simulink model "AC_Overall"  (R2021b)
settings: Solver=VariableStepAuto  StartTime=0.0  StopTime=0.5  RelTol=1e-3
undefined symbols (not defined in the file): ac
libraries: acoustical_lib x129, nesl_utility x4
(part 2 of 3)

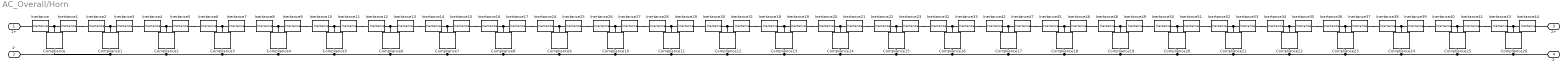
== system AC_Overall/Horn ==
  Compliance : acoustical_lib/Acoustical Elements/Compliance  c=ac.ho.C(1) m^3/Pa  r_c=1e-12 Pa/(m^3/s)  g_c=0 m^3/(Pa*s)  u_specify=off  u_priority=None  u=0 m^3/s  u_nominal_specify=off  u_nominal_unit=m^3/s  u_nominal_value=1  p_specify=off  p_priority=None  p=0 Pa  p_nominal_specify=off  p_nominal_unit=Pa  p_nominal_value=1  Pc_specify=off  Pc_priority=High  Pc=0 Pa  Pc_nominal_specify=off  Pc_nominal_unit=Pa  Pc_nominal_value=1
      settings: SourceProductName=Acoustical  InternalSimscapePortConfiguration="{\"Bottom\":[],\"Left\":[{\"id\":\"pp\",\"label\":\"+\",\"type\":\"acoustical.acoustical\"}],\"Right\":[{\"id\":\"nn\",\"label\":\"-\",\"type\":\"acoustical.acoustical\"}],\"Top\":[]}"
  Compliance1 : acoustical_lib/Acoustical Elements/Compliance  c=ac.ho.C(2) m^3/Pa  r_c=1e-12 Pa/(m^3/s)  g_c=0 m^3/(Pa*s)  u_specify=off  u_priority=None  u=0 m^3/s  u_nominal_specify=off  u_nominal_unit=m^3/s  u_nominal_value=1  p_specify=off  p_priority=None  p=0 Pa  p_nominal_specify=off  p_nominal_unit=Pa  p_nominal_value=1  Pc_specify=off  Pc_priority=High  Pc=0 Pa  Pc_nominal_specify=off  Pc_nominal_unit=Pa  Pc_nominal_value=1
      settings: SourceProductName=Acoustical  InternalSimscapePortConfiguration="{\"Bottom\":[],\"Left\":[{\"id\":\"pp\",\"label\":\"+\",\"type\":\"acoustical.acoustical\"}],\"Right\":[{\"id\":\"nn\",\"label\":\"-\",\"type\":\"acoustical.acoustical\"}],\"Top\":[]}"
  Compliance10 : acoustical_lib/Acoustical Elements/Compliance  c=ac.ho.C(11) m^3/Pa  r_c=1e-12 Pa/(m^3/s)  g_c=0 m^3/(Pa*s)  u_specify=off  u_priority=None  u=0 m^3/s  u_nominal_specify=off  u_nominal_unit=m^3/s  u_nominal_value=1  p_specify=off  p_priority=None  p=0 Pa  p_nominal_specify=off  p_nominal_unit=Pa  p_nominal_value=1  Pc_specify=off  Pc_priority=High  Pc=0 Pa  Pc_nominal_specify=off  Pc_nominal_unit=Pa  Pc_nominal_value=1
      settings: SourceProductName=Acoustical  InternalSimscapePortConfiguration="{\"Bottom\":[],\"Left\":[{\"id\":\"pp\",\"label\":\"+\",\"type\":\"acoustical.acoustical\"}],\"Right\":[{\"id\":\"nn\",\"label\":\"-\",\"type\":\"acoustical.acoustical\"}],\"Top\":[]}"
  Compliance11 : acoustical_lib/Acoustical Elements/Compliance  c=ac.ho.C(12) m^3/Pa  r_c=1e-12 Pa/(m^3/s)  g_c=0 m^3/(Pa*s)  u_specify=off  u_priority=None  u=0 m^3/s  u_nominal_specify=off  u_nominal_unit=m^3/s  u_nominal_value=1  p_specify=off  p_priority=None  p=0 Pa  p_nominal_specify=off  p_nominal_unit=Pa  p_nominal_value=1  Pc_specify=off  Pc_priority=High  Pc=0 Pa  Pc_nominal_specify=off  Pc_nominal_unit=Pa  Pc_nominal_value=1
      settings: SourceProductName=Acoustical  InternalSimscapePortConfiguration="{\"Bottom\":[],\"Left\":[{\"id\":\"pp\",\"label\":\"+\",\"type\":\"acoustical.acoustical\"}],\"Right\":[{\"id\":\"nn\",\"label\":\"-\",\"type\":\"acoustical.acoustical\"}],\"Top\":[]}"
  Compliance12 : acoustical_lib/Acoustical Elements/Compliance  c=ac.ho.C(13) m^3/Pa  r_c=1e-12 Pa/(m^3/s)  g_c=0 m^3/(Pa*s)  u_specify=off  u_priority=None  u=0 m^3/s  u_nominal_specify=off  u_nominal_unit=m^3/s  u_nominal_value=1  p_specify=off  p_priority=None  p=0 Pa  p_nominal_specify=off  p_nominal_unit=Pa  p_nominal_value=1  Pc_specify=off  Pc_priority=High  Pc=0 Pa  Pc_nominal_specify=off  Pc_nominal_unit=Pa  Pc_nominal_value=1
      settings: SourceProductName=Acoustical  InternalSimscapePortConfiguration="{\"Bottom\":[],\"Left\":[{\"id\":\"pp\",\"label\":\"+\",\"type\":\"acoustical.acoustical\"}],\"Right\":[{\"id\":\"nn\",\"label\":\"-\",\"type\":\"acoustical.acoustical\"}],\"Top\":[]}"
  Compliance13 : acoustical_lib/Acoustical Elements/Compliance  c=ac.ho.C(14) m^3/Pa  r_c=1e-12 Pa/(m^3/s)  g_c=0 m^3/(Pa*s)  u_specify=off  u_priority=None  u=0 m^3/s  u_nominal_specify=off  u_nominal_unit=m^3/s  u_nominal_value=1  p_specify=off  p_priority=None  p=0 Pa  p_nominal_specify=off  p_nominal_unit=Pa  p_nominal_value=1  Pc_specify=off  Pc_priority=High  Pc=0 Pa  Pc_nominal_specify=off  Pc_nominal_unit=Pa  Pc_nominal_value=1
      settings: SourceProductName=Acoustical  InternalSimscapePortConfiguration="{\"Bottom\":[],\"Left\":[{\"id\":\"pp\",\"label\":\"+\",\"type\":\"acoustical.acoustical\"}],\"Right\":[{\"id\":\"nn\",\"label\":\"-\",\"type\":\"acoustical.acoustical\"}],\"Top\":[]}"
  Compliance14 : acoustical_lib/Acoustical Elements/Compliance  c=ac.ho.C(15) m^3/Pa  r_c=1e-12 Pa/(m^3/s)  g_c=0 m^3/(Pa*s)  u_specify=off  u_priority=None  u=0 m^3/s  u_nominal_specify=off  u_nominal_unit=m^3/s  u_nominal_value=1  p_specify=off  p_priority=None  p=0 Pa  p_nominal_specify=off  p_nominal_unit=Pa  p_nominal_value=1  Pc_specify=off  Pc_priority=High  Pc=0 Pa  Pc_nominal_specify=off  Pc_nominal_unit=Pa  Pc_nominal_value=1
      settings: SourceProductName=Acoustical  InternalSimscapePortConfiguration="{\"Bottom\":[],\"Left\":[{\"id\":\"pp\",\"label\":\"+\",\"type\":\"acoustical.acoustical\"}],\"Right\":[{\"id\":\"nn\",\"label\":\"-\",\"type\":\"acoustical.acoustical\"}],\"Top\":[]}"
  Compliance15 : acoustical_lib/Acoustical Elements/Compliance  c=ac.ho.C(16) m^3/Pa  r_c=1e-12 Pa/(m^3/s)  g_c=0 m^3/(Pa*s)  u_specify=off  u_priority=None  u=0 m^3/s  u_nominal_specify=off  u_nominal_unit=m^3/s  u_nominal_value=1  p_specify=off  p_priority=None  p=0 Pa  p_nominal_specify=off  p_nominal_unit=Pa  p_nominal_value=1  Pc_specify=off  Pc_priority=High  Pc=0 Pa  Pc_nominal_specify=off  Pc_nominal_unit=Pa  Pc_nominal_value=1
      settings: SourceProductName=Acoustical  InternalSimscapePortConfiguration="{\"Bottom\":[],\"Left\":[{\"id\":\"pp\",\"label\":\"+\",\"type\":\"acoustical.acoustical\"}],\"Right\":[{\"id\":\"nn\",\"label\":\"-\",\"type\":\"acoustical.acoustical\"}],\"Top\":[]}"
  Compliance16 : acoustical_lib/Acoustical Elements/Compliance  c=ac.ho.C(17) m^3/Pa  r_c=1e-12 Pa/(m^3/s)  g_c=0 m^3/(Pa*s)  u_specify=off  u_priority=None  u=0 m^3/s  u_nominal_specify=off  u_nominal_unit=m^3/s  u_nominal_value=1  p_specify=off  p_priority=None  p=0 Pa  p_nominal_specify=off  p_nominal_unit=Pa  p_nominal_value=1  Pc_specify=off  Pc_priority=High  Pc=0 Pa  Pc_nominal_specify=off  Pc_nominal_unit=Pa  Pc_nominal_value=1
      settings: SourceProductName=Acoustical  InternalSimscapePortConfiguration="{\"Bottom\":[],\"Left\":[{\"id\":\"pp\",\"label\":\"+\",\"type\":\"acoustical.acoustical\"}],\"Right\":[{\"id\":\"nn\",\"label\":\"-\",\"type\":\"acoustical.acoustical\"}],\"Top\":[]}"
  Compliance17 : acoustical_lib/Acoustical Elements/Compliance  c=ac.ho.C(18) m^3/Pa  r_c=1e-12 Pa/(m^3/s)  g_c=0 m^3/(Pa*s)  u_specify=off  u_priority=None  u=0 m^3/s  u_nominal_specify=off  u_nominal_unit=m^3/s  u_nominal_value=1  p_specify=off  p_priority=None  p=0 Pa  p_nominal_specify=off  p_nominal_unit=Pa  p_nominal_value=1  Pc_specify=off  Pc_priority=High  Pc=0 Pa  Pc_nominal_specify=off  Pc_nominal_unit=Pa  Pc_nominal_value=1
      settings: SourceProductName=Acoustical  InternalSimscapePortConfiguration="{\"Bottom\":[],\"Left\":[{\"id\":\"pp\",\"label\":\"+\",\"type\":\"acoustical.acoustical\"}],\"Right\":[{\"id\":\"nn\",\"label\":\"-\",\"type\":\"acoustical.acoustical\"}],\"Top\":[]}"
  Compliance18 : acoustical_lib/Acoustical Elements/Compliance  c=ac.ho.C(19) m^3/Pa  r_c=1e-12 Pa/(m^3/s)  g_c=0 m^3/(Pa*s)  u_specify=off  u_priority=None  u=0 m^3/s  u_nominal_specify=off  u_nominal_unit=m^3/s  u_nominal_value=1  p_specify=off  p_priority=None  p=0 Pa  p_nominal_specify=off  p_nominal_unit=Pa  p_nominal_value=1  Pc_specify=off  Pc_priority=High  Pc=0 Pa  Pc_nominal_specify=off  Pc_nominal_unit=Pa  Pc_nominal_value=1
      settings: SourceProductName=Acoustical  InternalSimscapePortConfiguration="{\"Bottom\":[],\"Left\":[{\"id\":\"pp\",\"label\":\"+\",\"type\":\"acoustical.acoustical\"}],\"Right\":[{\"id\":\"nn\",\"label\":\"-\",\"type\":\"acoustical.acoustical\"}],\"Top\":[]}"
  Compliance19 : acoustical_lib/Acoustical Elements/Compliance  c=ac.ho.C(20) m^3/Pa  r_c=1e-12 Pa/(m^3/s)  g_c=0 m^3/(Pa*s)  u_specify=off  u_priority=None  u=0 m^3/s  u_nominal_specify=off  u_nominal_unit=m^3/s  u_nominal_value=1  p_specify=off  p_priority=None  p=0 Pa  p_nominal_specify=off  p_nominal_unit=Pa  p_nominal_value=1  Pc_specify=off  Pc_priority=High  Pc=0 Pa  Pc_nominal_specify=off  Pc_nominal_unit=Pa  Pc_nominal_value=1
      settings: SourceProductName=Acoustical  InternalSimscapePortConfiguration="{\"Bottom\":[],\"Left\":[{\"id\":\"pp\",\"label\":\"+\",\"type\":\"acoustical.acoustical\"}],\"Right\":[{\"id\":\"nn\",\"label\":\"-\",\"type\":\"acoustical.acoustical\"}],\"Top\":[]}"
  Compliance2 : acoustical_lib/Acoustical Elements/Compliance  c=ac.ho.C(3) m^3/Pa  r_c=1e-12 Pa/(m^3/s)  g_c=0 m^3/(Pa*s)  u_specify=off  u_priority=None  u=0 m^3/s  u_nominal_specify=off  u_nominal_unit=m^3/s  u_nominal_value=1  p_specify=off  p_priority=None  p=0 Pa  p_nominal_specify=off  p_nominal_unit=Pa  p_nominal_value=1  Pc_specify=off  Pc_priority=High  Pc=0 Pa  Pc_nominal_specify=off  Pc_nominal_unit=Pa  Pc_nominal_value=1
      settings: SourceProductName=Acoustical  InternalSimscapePortConfiguration="{\"Bottom\":[],\"Left\":[{\"id\":\"pp\",\"label\":\"+\",\"type\":\"acoustical.acoustical\"}],\"Right\":[{\"id\":\"nn\",\"label\":\"-\",\"type\":\"acoustical.acoustical\"}],\"Top\":[]}"
  Compliance20 : acoustical_lib/Acoustical Elements/Compliance  c=ac.ho.C(21) m^3/Pa  r_c=1e-12 Pa/(m^3/s)  g_c=0 m^3/(Pa*s)  u_specify=off  u_priority=None  u=0 m^3/s  u_nominal_specify=off  u_nominal_unit=m^3/s  u_nominal_value=1  p_specify=off  p_priority=None  p=0 Pa  p_nominal_specify=off  p_nominal_unit=Pa  p_nominal_value=1  Pc_specify=off  Pc_priority=High  Pc=0 Pa  Pc_nominal_specify=off  Pc_nominal_unit=Pa  Pc_nominal_value=1
      settings: SourceProductName=Acoustical  InternalSimscapePortConfiguration="{\"Bottom\":[],\"Left\":[{\"id\":\"pp\",\"label\":\"+\",\"type\":\"acoustical.acoustical\"}],\"Right\":[{\"id\":\"nn\",\"label\":\"-\",\"type\":\"acoustical.acoustical\"}],\"Top\":[]}"
  Compliance21 : acoustical_lib/Acoustical Elements/Compliance  c=ac.ho.C(22) m^3/Pa  r_c=1e-12 Pa/(m^3/s)  g_c=0 m^3/(Pa*s)  u_specify=off  u_priority=None  u=0 m^3/s  u_nominal_specify=off  u_nominal_unit=m^3/s  u_nominal_value=1  p_specify=off  p_priority=None  p=0 Pa  p_nominal_specify=off  p_nominal_unit=Pa  p_nominal_value=1  Pc_specify=off  Pc_priority=High  Pc=0 Pa  Pc_nominal_specify=off  Pc_nominal_unit=Pa  Pc_nominal_value=1
      settings: SourceProductName=Acoustical  InternalSimscapePortConfiguration="{\"Bottom\":[],\"Left\":[{\"id\":\"pp\",\"label\":\"+\",\"type\":\"acoustical.acoustical\"}],\"Right\":[{\"id\":\"nn\",\"label\":\"-\",\"type\":\"acoustical.acoustical\"}],\"Top\":[]}"
  Compliance22 : acoustical_lib/Acoustical Elements/Compliance  c=ac.ho.C(23) m^3/Pa  r_c=1e-12 Pa/(m^3/s)  g_c=0 m^3/(Pa*s)  u_specify=off  u_priority=None  u=0 m^3/s  u_nominal_specify=off  u_nominal_unit=m^3/s  u_nominal_value=1  p_specify=off  p_priority=None  p=0 Pa  p_nominal_specify=off  p_nominal_unit=Pa  p_nominal_value=1  Pc_specify=off  Pc_priority=High  Pc=0 Pa  Pc_nominal_specify=off  Pc_nominal_unit=Pa  Pc_nominal_value=1
      settings: SourceProductName=Acoustical  InternalSimscapePortConfiguration="{\"Bottom\":[],\"Left\":[{\"id\":\"pp\",\"label\":\"+\",\"type\":\"acoustical.acoustical\"}],\"Right\":[{\"id\":\"nn\",\"label\":\"-\",\"type\":\"acoustical.acoustical\"}],\"Top\":[]}"
  Compliance23 : acoustical_lib/Acoustical Elements/Compliance  c=ac.ho.C(24) m^3/Pa  r_c=1e-12 Pa/(m^3/s)  g_c=0 m^3/(Pa*s)  u_specify=off  u_priority=None  u=0 m^3/s  u_nominal_specify=off  u_nominal_unit=m^3/s  u_nominal_value=1  p_specify=off  p_priority=None  p=0 Pa  p_nominal_specify=off  p_nominal_unit=Pa  p_nominal_value=1  Pc_specify=off  Pc_priority=High  Pc=0 Pa  Pc_nominal_specify=off  Pc_nominal_unit=Pa  Pc_nominal_value=1
      settings: SourceProductName=Acoustical  InternalSimscapePortConfiguration="{\"Bottom\":[],\"Left\":[{\"id\":\"pp\",\"label\":\"+\",\"type\":\"acoustical.acoustical\"}],\"Right\":[{\"id\":\"nn\",\"label\":\"-\",\"type\":\"acoustical.acoustical\"}],\"Top\":[]}"
  Compliance24 : acoustical_lib/Acoustical Elements/Compliance  c=ac.ho.C(25) m^3/Pa  r_c=1e-12 Pa/(m^3/s)  g_c=0 m^3/(Pa*s)  u_specify=off  u_priority=None  u=0 m^3/s  u_nominal_specify=off  u_nominal_unit=m^3/s  u_nominal_value=1  p_specify=off  p_priority=None  p=0 Pa  p_nominal_specify=off  p_nominal_unit=Pa  p_nominal_value=1  Pc_specify=off  Pc_priority=High  Pc=0 Pa  Pc_nominal_specify=off  Pc_nominal_unit=Pa  Pc_nominal_value=1
      settings: SourceProductName=Acoustical  InternalSimscapePortConfiguration="{\"Bottom\":[],\"Left\":[{\"id\":\"pp\",\"label\":\"+\",\"type\":\"acoustical.acoustical\"}],\"Right\":[{\"id\":\"nn\",\"label\":\"-\",\"type\":\"acoustical.acoustical\"}],\"Top\":[]}"
  Compliance25 : acoustical_lib/Acoustical Elements/Compliance  c=ac.ho.C(26) m^3/Pa  r_c=1e-12 Pa/(m^3/s)  g_c=0 m^3/(Pa*s)  u_specify=off  u_priority=None  u=0 m^3/s  u_nominal_specify=off  u_nominal_unit=m^3/s  u_nominal_value=1  p_specify=off  p_priority=None  p=0 Pa  p_nominal_specify=off  p_nominal_unit=Pa  p_nominal_value=1  Pc_specify=off  Pc_priority=High  Pc=0 Pa  Pc_nominal_specify=off  Pc_nominal_unit=Pa  Pc_nominal_value=1
      settings: SourceProductName=Acoustical  InternalSimscapePortConfiguration="{\"Bottom\":[],\"Left\":[{\"id\":\"pp\",\"label\":\"+\",\"type\":\"acoustical.acoustical\"}],\"Right\":[{\"id\":\"nn\",\"label\":\"-\",\"type\":\"acoustical.acoustical\"}],\"Top\":[]}"
  Compliance26 : acoustical_lib/Acoustical Elements/Compliance  c=ac.ho.C(27) m^3/Pa  r_c=1e-12 Pa/(m^3/s)  g_c=0 m^3/(Pa*s)  u_specify=off  u_priority=None  u=0 m^3/s  u_nominal_specify=off  u_nominal_unit=m^3/s  u_nominal_value=1  p_specify=off  p_priority=None  p=0 Pa  p_nominal_specify=off  p_nominal_unit=Pa  p_nominal_value=1  Pc_specify=off  Pc_priority=High  Pc=0 Pa  Pc_nominal_specify=off  Pc_nominal_unit=Pa  Pc_nominal_value=1
      settings: SourceProductName=Acoustical  InternalSimscapePortConfiguration="{\"Bottom\":[],\"Left\":[{\"id\":\"pp\",\"label\":\"+\",\"type\":\"acoustical.acoustical\"}],\"Right\":[{\"id\":\"nn\",\"label\":\"-\",\"type\":\"acoustical.acoustical\"}],\"Top\":[]}"
  Compliance3 : acoustical_lib/Acoustical Elements/Compliance  c=ac.ho.C(4) m^3/Pa  r_c=1e-12 Pa/(m^3/s)  g_c=0 m^3/(Pa*s)  u_specify=off  u_priority=None  u=0 m^3/s  u_nominal_specify=off  u_nominal_unit=m^3/s  u_nominal_value=1  p_specify=off  p_priority=None  p=0 Pa  p_nominal_specify=off  p_nominal_unit=Pa  p_nominal_value=1  Pc_specify=off  Pc_priority=High  Pc=0 Pa  Pc_nominal_specify=off  Pc_nominal_unit=Pa  Pc_nominal_value=1
      settings: SourceProductName=Acoustical  InternalSimscapePortConfiguration="{\"Bottom\":[],\"Left\":[{\"id\":\"pp\",\"label\":\"+\",\"type\":\"acoustical.acoustical\"}],\"Right\":[{\"id\":\"nn\",\"label\":\"-\",\"type\":\"acoustical.acoustical\"}],\"Top\":[]}"
  Compliance4 : acoustical_lib/Acoustical Elements/Compliance  c=ac.ho.C(5) m^3/Pa  r_c=1e-12 Pa/(m^3/s)  g_c=0 m^3/(Pa*s)  u_specify=off  u_priority=None  u=0 m^3/s  u_nominal_specify=off  u_nominal_unit=m^3/s  u_nominal_value=1  p_specify=off  p_priority=None  p=0 Pa  p_nominal_specify=off  p_nominal_unit=Pa  p_nominal_value=1  Pc_specify=off  Pc_priority=High  Pc=0 Pa  Pc_nominal_specify=off  Pc_nominal_unit=Pa  Pc_nominal_value=1
      settings: SourceProductName=Acoustical  InternalSimscapePortConfiguration="{\"Bottom\":[],\"Left\":[{\"id\":\"pp\",\"label\":\"+\",\"type\":\"acoustical.acoustical\"}],\"Right\":[{\"id\":\"nn\",\"label\":\"-\",\"type\":\"acoustical.acoustical\"}],\"Top\":[]}"
  Compliance5 : acoustical_lib/Acoustical Elements/Compliance  c=ac.ho.C(6) m^3/Pa  r_c=1e-12 Pa/(m^3/s)  g_c=0 m^3/(Pa*s)  u_specify=off  u_priority=None  u=0 m^3/s  u_nominal_specify=off  u_nominal_unit=m^3/s  u_nominal_value=1  p_specify=off  p_priority=None  p=0 Pa  p_nominal_specify=off  p_nominal_unit=Pa  p_nominal_value=1  Pc_specify=off  Pc_priority=High  Pc=0 Pa  Pc_nominal_specify=off  Pc_nominal_unit=Pa  Pc_nominal_value=1
      settings: SourceProductName=Acoustical  InternalSimscapePortConfiguration="{\"Bottom\":[],\"Left\":[{\"id\":\"pp\",\"label\":\"+\",\"type\":\"acoustical.acoustical\"}],\"Right\":[{\"id\":\"nn\",\"label\":\"-\",\"type\":\"acoustical.acoustical\"}],\"Top\":[]}"
  Compliance6 : acoustical_lib/Acoustical Elements/Compliance  c=ac.ho.C(7) m^3/Pa  r_c=1e-12 Pa/(m^3/s)  g_c=0 m^3/(Pa*s)  u_specify=off  u_priority=None  u=0 m^3/s  u_nominal_specify=off  u_nominal_unit=m^3/s  u_nominal_value=1  p_specify=off  p_priority=None  p=0 Pa  p_nominal_specify=off  p_nominal_unit=Pa  p_nominal_value=1  Pc_specify=off  Pc_priority=High  Pc=0 Pa  Pc_nominal_specify=off  Pc_nominal_unit=Pa  Pc_nominal_value=1
      settings: SourceProductName=Acoustical  InternalSimscapePortConfiguration="{\"Bottom\":[],\"Left\":[{\"id\":\"pp\",\"label\":\"+\",\"type\":\"acoustical.acoustical\"}],\"Right\":[{\"id\":\"nn\",\"label\":\"-\",\"type\":\"acoustical.acoustical\"}],\"Top\":[]}"
  Compliance7 : acoustical_lib/Acoustical Elements/Compliance  c=ac.ho.C(8) m^3/Pa  r_c=1e-12 Pa/(m^3/s)  g_c=0 m^3/(Pa*s)  u_specify=off  u_priority=None  u=0 m^3/s  u_nominal_specify=off  u_nominal_unit=m^3/s  u_nominal_value=1  p_specify=off  p_priority=None  p=0 Pa  p_nominal_specify=off  p_nominal_unit=Pa  p_nominal_value=1  Pc_specify=off  Pc_priority=High  Pc=0 Pa  Pc_nominal_specify=off  Pc_nominal_unit=Pa  Pc_nominal_value=1
      settings: SourceProductName=Acoustical  InternalSimscapePortConfiguration="{\"Bottom\":[],\"Left\":[{\"id\":\"pp\",\"label\":\"+\",\"type\":\"acoustical.acoustical\"}],\"Right\":[{\"id\":\"nn\",\"label\":\"-\",\"type\":\"acoustical.acoustical\"}],\"Top\":[]}"
  Compliance8 : acoustical_lib/Acoustical Elements/Compliance  c=ac.ho.C(9) m^3/Pa  r_c=1e-12 Pa/(m^3/s)  g_c=0 m^3/(Pa*s)  u_specify=off  u_priority=None  u=0 m^3/s  u_nominal_specify=off  u_nominal_unit=m^3/s  u_nominal_value=1  p_specify=off  p_priority=None  p=0 Pa  p_nominal_specify=off  p_nominal_unit=Pa  p_nominal_value=1  Pc_specify=off  Pc_priority=High  Pc=0 Pa  Pc_nominal_specify=off  Pc_nominal_unit=Pa  Pc_nominal_value=1
      settings: SourceProductName=Acoustical  InternalSimscapePortConfiguration="{\"Bottom\":[],\"Left\":[{\"id\":\"pp\",\"label\":\"+\",\"type\":\"acoustical.acoustical\"}],\"Right\":[{\"id\":\"nn\",\"label\":\"-\",\"type\":\"acoustical.acoustical\"}],\"Top\":[]}"
  Compliance9 : acoustical_lib/Acoustical Elements/Compliance  c=ac.ho.C(10) m^3/Pa  r_c=1e-12 Pa/(m^3/s)  g_c=0 m^3/(Pa*s)  u_specify=off  u_priority=None  u=0 m^3/s  u_nominal_specify=off  u_nominal_unit=m^3/s  u_nominal_value=1  p_specify=off  p_priority=None  p=0 Pa  p_nominal_specify=off  p_nominal_unit=Pa  p_nominal_value=1  Pc_specify=off  Pc_priority=High  Pc=0 Pa  Pc_nominal_specify=off  Pc_nominal_unit=Pa  Pc_nominal_value=1
      settings: SourceProductName=Acoustical  InternalSimscapePortConfiguration="{\"Bottom\":[],\"Left\":[{\"id\":\"pp\",\"label\":\"+\",\"type\":\"acoustical.acoustical\"}],\"Right\":[{\"id\":\"nn\",\"label\":\"-\",\"type\":\"acoustical.acoustical\"}],\"Top\":[]}"
  Inertance : acoustical_lib/Acoustical Elements/Inertance  m=ac.ho.L(1) Pa*s^2/m^3  r_m=0 Pa/(m^3/s)  g_m=1e-12 m^3/(Pa*s)  u_specify=off  u_priority=None  u=0 m^3/s  u_nominal_specify=off  u_nominal_unit=m^3/s  u_nominal_value=1  p_specify=off  p_priority=None  p=0 Pa  p_nominal_specify=off  p_nominal_unit=Pa  p_nominal_value=1  U_m_specify=off  U_m_priority=High  U_m=0 m^3/s  U_m_nominal_specify=off  U_m_nominal_unit=m^3/s  U_m_nominal_value=1
      settings: SourceProductName=Acoustical  InternalSimscapePortConfiguration="{\"Bottom\":[],\"Left\":[{\"id\":\"pp\",\"label\":\"+\",\"type\":\"acoustical.acoustical\"}],\"Right\":[{\"id\":\"nn\",\"label\":\"-\",\"type\":\"acoustical.acoustical\"}],\"Top\":[]}"
  Inertance1 : acoustical_lib/Acoustical Elements/Inertance  m=ac.ho.L(1) Pa*s^2/m^3  r_m=0 Pa/(m^3/s)  g_m=1e-12 m^3/(Pa*s)  u_specify=off  u_priority=None  u=0 m^3/s  u_nominal_specify=off  u_nominal_unit=m^3/s  u_nominal_value=1  p_specify=off  p_priority=None  p=0 Pa  p_nominal_specify=off  p_nominal_unit=Pa  p_nominal_value=1  U_m_specify=off  U_m_priority=High  U_m=0 m^3/s  U_m_nominal_specify=off  U_m_nominal_unit=m^3/s  U_m_nominal_value=1
      settings: SourceProductName=Acoustical  InternalSimscapePortConfiguration="{\"Bottom\":[],\"Left\":[{\"id\":\"pp\",\"label\":\"+\",\"type\":\"acoustical.acoustical\"}],\"Right\":[{\"id\":\"nn\",\"label\":\"-\",\"type\":\"acoustical.acoustical\"}],\"Top\":[]}"
  Inertance10 : acoustical_lib/Acoustical Elements/Inertance  m=ac.ho.L(6) Pa*s^2/m^3  r_m=0 Pa/(m^3/s)  g_m=1e-12 m^3/(Pa*s)  u_specify=off  u_priority=None  u=0 m^3/s  u_nominal_specify=off  u_nominal_unit=m^3/s  u_nominal_value=1  p_specify=off  p_priority=None  p=0 Pa  p_nominal_specify=off  p_nominal_unit=Pa  p_nominal_value=1  U_m_specify=off  U_m_priority=High  U_m=0 m^3/s  U_m_nominal_specify=off  U_m_nominal_unit=m^3/s  U_m_nominal_value=1
      settings: SourceProductName=Acoustical  InternalSimscapePortConfiguration="{\"Bottom\":[],\"Left\":[{\"id\":\"pp\",\"label\":\"+\",\"type\":\"acoustical.acoustical\"}],\"Right\":[{\"id\":\"nn\",\"label\":\"-\",\"type\":\"acoustical.acoustical\"}],\"Top\":[]}"
  Inertance11 : acoustical_lib/Acoustical Elements/Inertance  m=ac.ho.L(6) Pa*s^2/m^3  r_m=0 Pa/(m^3/s)  g_m=1e-12 m^3/(Pa*s)  u_specify=off  u_priority=None  u=0 m^3/s  u_nominal_specify=off  u_nominal_unit=m^3/s  u_nominal_value=1  p_specify=off  p_priority=None  p=0 Pa  p_nominal_specify=off  p_nominal_unit=Pa  p_nominal_value=1  U_m_specify=off  U_m_priority=High  U_m=0 m^3/s  U_m_nominal_specify=off  U_m_nominal_unit=m^3/s  U_m_nominal_value=1
      settings: SourceProductName=Acoustical  InternalSimscapePortConfiguration="{\"Bottom\":[],\"Left\":[{\"id\":\"pp\",\"label\":\"+\",\"type\":\"acoustical.acoustical\"}],\"Right\":[{\"id\":\"nn\",\"label\":\"-\",\"type\":\"acoustical.acoustical\"}],\"Top\":[]}"
  Inertance12 : acoustical_lib/Acoustical Elements/Inertance  m=ac.ho.L(7) Pa*s^2/m^3  r_m=0 Pa/(m^3/s)  g_m=1e-12 m^3/(Pa*s)  u_specify=off  u_priority=None  u=0 m^3/s  u_nominal_specify=off  u_nominal_unit=m^3/s  u_nominal_value=1  p_specify=off  p_priority=None  p=0 Pa  p_nominal_specify=off  p_nominal_unit=Pa  p_nominal_value=1  U_m_specify=off  U_m_priority=High  U_m=0 m^3/s  U_m_nominal_specify=off  U_m_nominal_unit=m^3/s  U_m_nominal_value=1
      settings: SourceProductName=Acoustical  InternalSimscapePortConfiguration="{\"Bottom\":[],\"Left\":[{\"id\":\"pp\",\"label\":\"+\",\"type\":\"acoustical.acoustical\"}],\"Right\":[{\"id\":\"nn\",\"label\":\"-\",\"type\":\"acoustical.acoustical\"}],\"Top\":[]}"
  Inertance13 : acoustical_lib/Acoustical Elements/Inertance  m=ac.ho.L(7) Pa*s^2/m^3  r_m=0 Pa/(m^3/s)  g_m=1e-12 m^3/(Pa*s)  u_specify=off  u_priority=None  u=0 m^3/s  u_nominal_specify=off  u_nominal_unit=m^3/s  u_nominal_value=1  p_specify=off  p_priority=None  p=0 Pa  p_nominal_specify=off  p_nominal_unit=Pa  p_nominal_value=1  U_m_specify=off  U_m_priority=High  U_m=0 m^3/s  U_m_nominal_specify=off  U_m_nominal_unit=m^3/s  U_m_nominal_value=1
      settings: SourceProductName=Acoustical  InternalSimscapePortConfiguration="{\"Bottom\":[],\"Left\":[{\"id\":\"pp\",\"label\":\"+\",\"type\":\"acoustical.acoustical\"}],\"Right\":[{\"id\":\"nn\",\"label\":\"-\",\"type\":\"acoustical.acoustical\"}],\"Top\":[]}"
  Inertance14 : acoustical_lib/Acoustical Elements/Inertance  m=ac.ho.L(8) Pa*s^2/m^3  r_m=0 Pa/(m^3/s)  g_m=1e-12 m^3/(Pa*s)  u_specify=off  u_priority=None  u=0 m^3/s  u_nominal_specify=off  u_nominal_unit=m^3/s  u_nominal_value=1  p_specify=off  p_priority=None  p=0 Pa  p_nominal_specify=off  p_nominal_unit=Pa  p_nominal_value=1  U_m_specify=off  U_m_priority=High  U_m=0 m^3/s  U_m_nominal_specify=off  U_m_nominal_unit=m^3/s  U_m_nominal_value=1
      settings: SourceProductName=Acoustical  InternalSimscapePortConfiguration="{\"Bottom\":[],\"Left\":[{\"id\":\"pp\",\"label\":\"+\",\"type\":\"acoustical.acoustical\"}],\"Right\":[{\"id\":\"nn\",\"label\":\"-\",\"type\":\"acoustical.acoustical\"}],\"Top\":[]}"
  Inertance15 : acoustical_lib/Acoustical Elements/Inertance  m=ac.ho.L(8) Pa*s^2/m^3  r_m=0 Pa/(m^3/s)  g_m=1e-12 m^3/(Pa*s)  u_specify=off  u_priority=None  u=0 m^3/s  u_nominal_specify=off  u_nominal_unit=m^3/s  u_nominal_value=1  p_specify=off  p_priority=None  p=0 Pa  p_nominal_specify=off  p_nominal_unit=Pa  p_nominal_value=1  U_m_specify=off  U_m_priority=High  U_m=0 m^3/s  U_m_nominal_specify=off  U_m_nominal_unit=m^3/s  U_m_nominal_value=1
      settings: SourceProductName=Acoustical  InternalSimscapePortConfiguration="{\"Bottom\":[],\"Left\":[{\"id\":\"pp\",\"label\":\"+\",\"type\":\"acoustical.acoustical\"}],\"Right\":[{\"id\":\"nn\",\"label\":\"-\",\"type\":\"acoustical.acoustical\"}],\"Top\":[]}"
  Inertance16 : acoustical_lib/Acoustical Elements/Inertance  m=ac.ho.L(9) Pa*s^2/m^3  r_m=0 Pa/(m^3/s)  g_m=1e-12 m^3/(Pa*s)  u_specify=off  u_priority=None  u=0 m^3/s  u_nominal_specify=off  u_nominal_unit=m^3/s  u_nominal_value=1  p_specify=off  p_priority=None  p=0 Pa  p_nominal_specify=off  p_nominal_unit=Pa  p_nominal_value=1  U_m_specify=off  U_m_priority=High  U_m=0 m^3/s  U_m_nominal_specify=off  U_m_nominal_unit=m^3/s  U_m_nominal_value=1
      settings: SourceProductName=Acoustical  InternalSimscapePortConfiguration="{\"Bottom\":[],\"Left\":[{\"id\":\"pp\",\"label\":\"+\",\"type\":\"acoustical.acoustical\"}],\"Right\":[{\"id\":\"nn\",\"label\":\"-\",\"type\":\"acoustical.acoustical\"}],\"Top\":[]}"
  Inertance17 : acoustical_lib/Acoustical Elements/Inertance  m=ac.ho.L(9) Pa*s^2/m^3  r_m=0 Pa/(m^3/s)  g_m=1e-12 m^3/(Pa*s)  u_specify=off  u_priority=None  u=0 m^3/s  u_nominal_specify=off  u_nominal_unit=m^3/s  u_nominal_value=1  p_specify=off  p_priority=None  p=0 Pa  p_nominal_specify=off  p_nominal_unit=Pa  p_nominal_value=1  U_m_specify=off  U_m_priority=High  U_m=0 m^3/s  U_m_nominal_specify=off  U_m_nominal_unit=m^3/s  U_m_nominal_value=1
      settings: SourceProductName=Acoustical  InternalSimscapePortConfiguration="{\"Bottom\":[],\"Left\":[{\"id\":\"pp\",\"label\":\"+\",\"type\":\"acoustical.acoustical\"}],\"Right\":[{\"id\":\"nn\",\"label\":\"-\",\"type\":\"acoustical.acoustical\"}],\"Top\":[]}"
  Inertance18 : acoustical_lib/Acoustical Elements/Inertance  m=ac.ho.L(14) Pa*s^2/m^3  r_m=0 Pa/(m^3/s)  g_m=1e-12 m^3/(Pa*s)  u_specify=off  u_priority=None  u=0 m^3/s  u_nominal_specify=off  u_nominal_unit=m^3/s  u_nominal_value=1  p_specify=off  p_priority=None  p=0 Pa  p_nominal_specify=off  p_nominal_unit=Pa  p_nominal_value=1  U_m_specify=off  U_m_priority=High  U_m=0 m^3/s  U_m_nominal_specify=off  U_m_nominal_unit=m^3/s  U_m_nominal_value=1
      settings: SourceProductName=Acoustical  InternalSimscapePortConfiguration="{\"Bottom\":[],\"Left\":[{\"id\":\"pp\",\"label\":\"+\",\"type\":\"acoustical.acoustical\"}],\"Right\":[{\"id\":\"nn\",\"label\":\"-\",\"type\":\"acoustical.acoustical\"}],\"Top\":[]}"
  Inertance19 : acoustical_lib/Acoustical Elements/Inertance  m=ac.ho.L(14) Pa*s^2/m^3  r_m=0 Pa/(m^3/s)  g_m=1e-12 m^3/(Pa*s)  u_specify=off  u_priority=None  u=0 m^3/s  u_nominal_specify=off  u_nominal_unit=m^3/s  u_nominal_value=1  p_specify=off  p_priority=None  p=0 Pa  p_nominal_specify=off  p_nominal_unit=Pa  p_nominal_value=1  U_m_specify=off  U_m_priority=High  U_m=0 m^3/s  U_m_nominal_specify=off  U_m_nominal_unit=m^3/s  U_m_nominal_value=1
      settings: SourceProductName=Acoustical  InternalSimscapePortConfiguration="{\"Bottom\":[],\"Left\":[{\"id\":\"pp\",\"label\":\"+\",\"type\":\"acoustical.acoustical\"}],\"Right\":[{\"id\":\"nn\",\"label\":\"-\",\"type\":\"acoustical.acoustical\"}],\"Top\":[]}"
  Inertance2 : acoustical_lib/Acoustical Elements/Inertance  m=ac.ho.L(2) Pa*s^2/m^3  r_m=0 Pa/(m^3/s)  g_m=1e-12 m^3/(Pa*s)  u_specify=off  u_priority=None  u=0 m^3/s  u_nominal_specify=off  u_nominal_unit=m^3/s  u_nominal_value=1  p_specify=off  p_priority=None  p=0 Pa  p_nominal_specify=off  p_nominal_unit=Pa  p_nominal_value=1  U_m_specify=off  U_m_priority=High  U_m=0 m^3/s  U_m_nominal_specify=off  U_m_nominal_unit=m^3/s  U_m_nominal_value=1
      settings: SourceProductName=Acoustical  InternalSimscapePortConfiguration="{\"Bottom\":[],\"Left\":[{\"id\":\"pp\",\"label\":\"+\",\"type\":\"acoustical.acoustical\"}],\"Right\":[{\"id\":\"nn\",\"label\":\"-\",\"type\":\"acoustical.acoustical\"}],\"Top\":[]}"
  Inertance20 : acoustical_lib/Acoustical Elements/Inertance  m=ac.ho.L(15) Pa*s^2/m^3  r_m=0 Pa/(m^3/s)  g_m=1e-12 m^3/(Pa*s)  u_specify=off  u_priority=None  u=0 m^3/s  u_nominal_specify=off  u_nominal_unit=m^3/s  u_nominal_value=1  p_specify=off  p_priority=None  p=0 Pa  p_nominal_specify=off  p_nominal_unit=Pa  p_nominal_value=1  U_m_specify=off  U_m_priority=High  U_m=0 m^3/s  U_m_nominal_specify=off  U_m_nominal_unit=m^3/s  U_m_nominal_value=1
      settings: SourceProductName=Acoustical  InternalSimscapePortConfiguration="{\"Bottom\":[],\"Left\":[{\"id\":\"pp\",\"label\":\"+\",\"type\":\"acoustical.acoustical\"}],\"Right\":[{\"id\":\"nn\",\"label\":\"-\",\"type\":\"acoustical.acoustical\"}],\"Top\":[]}"
  Inertance21 : acoustical_lib/Acoustical Elements/Inertance  m=ac.ho.L(15) Pa*s^2/m^3  r_m=0 Pa/(m^3/s)  g_m=1e-12 m^3/(Pa*s)  u_specify=off  u_priority=None  u=0 m^3/s  u_nominal_specify=off  u_nominal_unit=m^3/s  u_nominal_value=1  p_specify=off  p_priority=None  p=0 Pa  p_nominal_specify=off  p_nominal_unit=Pa  p_nominal_value=1  U_m_specify=off  U_m_priority=High  U_m=0 m^3/s  U_m_nominal_specify=off  U_m_nominal_unit=m^3/s  U_m_nominal_value=1
      settings: SourceProductName=Acoustical  InternalSimscapePortConfiguration="{\"Bottom\":[],\"Left\":[{\"id\":\"pp\",\"label\":\"+\",\"type\":\"acoustical.acoustical\"}],\"Right\":[{\"id\":\"nn\",\"label\":\"-\",\"type\":\"acoustical.acoustical\"}],\"Top\":[]}"
  Inertance22 : acoustical_lib/Acoustical Elements/Inertance  m=ac.ho.L(16) Pa*s^2/m^3  r_m=0 Pa/(m^3/s)  g_m=1e-12 m^3/(Pa*s)  u_specify=off  u_priority=None  u=0 m^3/s  u_nominal_specify=off  u_nominal_unit=m^3/s  u_nominal_value=1  p_specify=off  p_priority=None  p=0 Pa  p_nominal_specify=off  p_nominal_unit=Pa  p_nominal_value=1  U_m_specify=off  U_m_priority=High  U_m=0 m^3/s  U_m_nominal_specify=off  U_m_nominal_unit=m^3/s  U_m_nominal_value=1
      settings: SourceProductName=Acoustical  InternalSimscapePortConfiguration="{\"Bottom\":[],\"Left\":[{\"id\":\"pp\",\"label\":\"+\",\"type\":\"acoustical.acoustical\"}],\"Right\":[{\"id\":\"nn\",\"label\":\"-\",\"type\":\"acoustical.acoustical\"}],\"Top\":[]}"
  Inertance23 : acoustical_lib/Acoustical Elements/Inertance  m=ac.ho.L(16) Pa*s^2/m^3  r_m=0 Pa/(m^3/s)  g_m=1e-12 m^3/(Pa*s)  u_specify=off  u_priority=None  u=0 m^3/s  u_nominal_specify=off  u_nominal_unit=m^3/s  u_nominal_value=1  p_specify=off  p_priority=None  p=0 Pa  p_nominal_specify=off  p_nominal_unit=Pa  p_nominal_value=1  U_m_specify=off  U_m_priority=High  U_m=0 m^3/s  U_m_nominal_specify=off  U_m_nominal_unit=m^3/s  U_m_nominal_value=1
      settings: SourceProductName=Acoustical  InternalSimscapePortConfiguration="{\"Bottom\":[],\"Left\":[{\"id\":\"pp\",\"label\":\"+\",\"type\":\"acoustical.acoustical\"}],\"Right\":[{\"id\":\"nn\",\"label\":\"-\",\"type\":\"acoustical.acoustical\"}],\"Top\":[]}"
  Inertance24 : acoustical_lib/Acoustical Elements/Inertance  m=ac.ho.L(10) Pa*s^2/m^3  r_m=0 Pa/(m^3/s)  g_m=1e-12 m^3/(Pa*s)  u_specify=off  u_priority=None  u=0 m^3/s  u_nominal_specify=off  u_nominal_unit=m^3/s  u_nominal_value=1  p_specify=off  p_priority=None  p=0 Pa  p_nominal_specify=off  p_nominal_unit=Pa  p_nominal_value=1  U_m_specify=off  U_m_priority=High  U_m=0 m^3/s  U_m_nominal_specify=off  U_m_nominal_unit=m^3/s  U_m_nominal_value=1
      settings: SourceProductName=Acoustical  InternalSimscapePortConfiguration="{\"Bottom\":[],\"Left\":[{\"id\":\"pp\",\"label\":\"+\",\"type\":\"acoustical.acoustical\"}],\"Right\":[{\"id\":\"nn\",\"label\":\"-\",\"type\":\"acoustical.acoustical\"}],\"Top\":[]}"
  Inertance25 : acoustical_lib/Acoustical Elements/Inertance  m=ac.ho.L(10) Pa*s^2/m^3  r_m=0 Pa/(m^3/s)  g_m=1e-12 m^3/(Pa*s)  u_specify=off  u_priority=None  u=0 m^3/s  u_nominal_specify=off  u_nominal_unit=m^3/s  u_nominal_value=1  p_specify=off  p_priority=None  p=0 Pa  p_nominal_specify=off  p_nominal_unit=Pa  p_nominal_value=1  U_m_specify=off  U_m_priority=High  U_m=0 m^3/s  U_m_nominal_specify=off  U_m_nominal_unit=m^3/s  U_m_nominal_value=1
      settings: SourceProductName=Acoustical  InternalSimscapePortConfiguration="{\"Bottom\":[],\"Left\":[{\"id\":\"pp\",\"label\":\"+\",\"type\":\"acoustical.acoustical\"}],\"Right\":[{\"id\":\"nn\",\"label\":\"-\",\"type\":\"acoustical.acoustical\"}],\"Top\":[]}"
  Inertance26 : acoustical_lib/Acoustical Elements/Inertance  m=ac.ho.L(11) Pa*s^2/m^3  r_m=0 Pa/(m^3/s)  g_m=1e-12 m^3/(Pa*s)  u_specify=off  u_priority=None  u=0 m^3/s  u_nominal_specify=off  u_nominal_unit=m^3/s  u_nominal_value=1  p_specify=off  p_priority=None  p=0 Pa  p_nominal_specify=off  p_nominal_unit=Pa  p_nominal_value=1  U_m_specify=off  U_m_priority=High  U_m=0 m^3/s  U_m_nominal_specify=off  U_m_nominal_unit=m^3/s  U_m_nominal_value=1
      settings: SourceProductName=Acoustical  InternalSimscapePortConfiguration="{\"Bottom\":[],\"Left\":[{\"id\":\"pp\",\"label\":\"+\",\"type\":\"acoustical.acoustical\"}],\"Right\":[{\"id\":\"nn\",\"label\":\"-\",\"type\":\"acoustical.acoustical\"}],\"Top\":[]}"
  Inertance27 : acoustical_lib/Acoustical Elements/Inertance  m=ac.ho.L(11) Pa*s^2/m^3  r_m=0 Pa/(m^3/s)  g_m=1e-12 m^3/(Pa*s)  u_specify=off  u_priority=None  u=0 m^3/s  u_nominal_specify=off  u_nominal_unit=m^3/s  u_nominal_value=1  p_specify=off  p_priority=None  p=0 Pa  p_nominal_specify=off  p_nominal_unit=Pa  p_nominal_value=1  U_m_specify=off  U_m_priority=High  U_m=0 m^3/s  U_m_nominal_specify=off  U_m_nominal_unit=m^3/s  U_m_nominal_value=1
      settings: SourceProductName=Acoustical  InternalSimscapePortConfiguration="{\"Bottom\":[],\"Left\":[{\"id\":\"pp\",\"label\":\"+\",\"type\":\"acoustical.acoustical\"}],\"Right\":[{\"id\":\"nn\",\"label\":\"-\",\"type\":\"acoustical.acoustical\"}],\"Top\":[]}"
  Inertance28 : acoustical_lib/Acoustical Elements/Inertance  m=ac.ho.L(12) Pa*s^2/m^3  r_m=0 Pa/(m^3/s)  g_m=1e-12 m^3/(Pa*s)  u_specify=off  u_priority=None  u=0 m^3/s  u_nominal_specify=off  u_nominal_unit=m^3/s  u_nominal_value=1  p_specify=off  p_priority=None  p=0 Pa  p_nominal_specify=off  p_nominal_unit=Pa  p_nominal_value=1  U_m_specify=off  U_m_priority=High  U_m=0 m^3/s  U_m_nominal_specify=off  U_m_nominal_unit=m^3/s  U_m_nominal_value=1
      settings: SourceProductName=Acoustical  InternalSimscapePortConfiguration="{\"Bottom\":[],\"Left\":[{\"id\":\"pp\",\"label\":\"+\",\"type\":\"acoustical.acoustical\"}],\"Right\":[{\"id\":\"nn\",\"label\":\"-\",\"type\":\"acoustical.acoustical\"}],\"Top\":[]}"
  Inertance29 : acoustical_lib/Acoustical Elements/Inertance  m=ac.ho.L(12) Pa*s^2/m^3  r_m=0 Pa/(m^3/s)  g_m=1e-12 m^3/(Pa*s)  u_specify=off  u_priority=None  u=0 m^3/s  u_nominal_specify=off  u_nominal_unit=m^3/s  u_nominal_value=1  p_specify=off  p_priority=None  p=0 Pa  p_nominal_specify=off  p_nominal_unit=Pa  p_nominal_value=1  U_m_specify=off  U_m_priority=High  U_m=0 m^3/s  U_m_nominal_specify=off  U_m_nominal_unit=m^3/s  U_m_nominal_value=1
      settings: SourceProductName=Acoustical  InternalSimscapePortConfiguration="{\"Bottom\":[],\"Left\":[{\"id\":\"pp\",\"label\":\"+\",\"type\":\"acoustical.acoustical\"}],\"Right\":[{\"id\":\"nn\",\"label\":\"-\",\"type\":\"acoustical.acoustical\"}],\"Top\":[]}"
  Inertance3 : acoustical_lib/Acoustical Elements/Inertance  m=ac.ho.L(2) Pa*s^2/m^3  r_m=0 Pa/(m^3/s)  g_m=1e-12 m^3/(Pa*s)  u_specify=off  u_priority=None  u=0 m^3/s  u_nominal_specify=off  u_nominal_unit=m^3/s  u_nominal_value=1  p_specify=off  p_priority=None  p=0 Pa  p_nominal_specify=off  p_nominal_unit=Pa  p_nominal_value=1  U_m_specify=off  U_m_priority=High  U_m=0 m^3/s  U_m_nominal_specify=off  U_m_nominal_unit=m^3/s  U_m_nominal_value=1
      settings: SourceProductName=Acoustical  InternalSimscapePortConfiguration="{\"Bottom\":[],\"Left\":[{\"id\":\"pp\",\"label\":\"+\",\"type\":\"acoustical.acoustical\"}],\"Right\":[{\"id\":\"nn\",\"label\":\"-\",\"type\":\"acoustical.acoustical\"}],\"Top\":[]}"
  Inertance30 : acoustical_lib/Acoustical Elements/Inertance  m=ac.ho.L(13) Pa*s^2/m^3  r_m=0 Pa/(m^3/s)  g_m=1e-12 m^3/(Pa*s)  u_specify=off  u_priority=None  u=0 m^3/s  u_nominal_specify=off  u_nominal_unit=m^3/s  u_nominal_value=1  p_specify=off  p_priority=None  p=0 Pa  p_nominal_specify=off  p_nominal_unit=Pa  p_nominal_value=1  U_m_specify=off  U_m_priority=High  U_m=0 m^3/s  U_m_nominal_specify=off  U_m_nominal_unit=m^3/s  U_m_nominal_value=1
      settings: SourceProductName=Acoustical  InternalSimscapePortConfiguration="{\"Bottom\":[],\"Left\":[{\"id\":\"pp\",\"label\":\"+\",\"type\":\"acoustical.acoustical\"}],\"Right\":[{\"id\":\"nn\",\"label\":\"-\",\"type\":\"acoustical.acoustical\"}],\"Top\":[]}"
  Inertance31 : acoustical_lib/Acoustical Elements/Inertance  m=ac.ho.L(13) Pa*s^2/m^3  r_m=0 Pa/(m^3/s)  g_m=1e-12 m^3/(Pa*s)  u_specify=off  u_priority=None  u=0 m^3/s  u_nominal_specify=off  u_nominal_unit=m^3/s  u_nominal_value=1  p_specify=off  p_priority=None  p=0 Pa  p_nominal_specify=off  p_nominal_unit=Pa  p_nominal_value=1  U_m_specify=off  U_m_priority=High  U_m=0 m^3/s  U_m_nominal_specify=off  U_m_nominal_unit=m^3/s  U_m_nominal_value=1
      settings: SourceProductName=Acoustical  InternalSimscapePortConfiguration="{\"Bottom\":[],\"Left\":[{\"id\":\"pp\",\"label\":\"+\",\"type\":\"acoustical.acoustical\"}],\"Right\":[{\"id\":\"nn\",\"label\":\"-\",\"type\":\"acoustical.acoustical\"}],\"Top\":[]}"
  Inertance32 : acoustical_lib/Acoustical Elements/Inertance  m=ac.ho.L(17) Pa*s^2/m^3  r_m=0 Pa/(m^3/s)  g_m=1e-12 m^3/(Pa*s)  u_specify=off  u_priority=None  u=0 m^3/s  u_nominal_specify=off  u_nominal_unit=m^3/s  u_nominal_value=1  p_specify=off  p_priority=None  p=0 Pa  p_nominal_specify=off  p_nominal_unit=Pa  p_nominal_value=1  U_m_specify=off  U_m_priority=High  U_m=0 m^3/s  U_m_nominal_specify=off  U_m_nominal_unit=m^3/s  U_m_nominal_value=1
      settings: SourceProductName=Acoustical  InternalSimscapePortConfiguration="{\"Bottom\":[],\"Left\":[{\"id\":\"pp\",\"label\":\"+\",\"type\":\"acoustical.acoustical\"}],\"Right\":[{\"id\":\"nn\",\"label\":\"-\",\"type\":\"acoustical.acoustical\"}],\"Top\":[]}"
  Inertance33 : acoustical_lib/Acoustical Elements/Inertance  m=ac.ho.L(17) Pa*s^2/m^3  r_m=0 Pa/(m^3/s)  g_m=1e-12 m^3/(Pa*s)  u_specify=off  u_priority=None  u=0 m^3/s  u_nominal_specify=off  u_nominal_unit=m^3/s  u_nominal_value=1  p_specify=off  p_priority=None  p=0 Pa  p_nominal_specify=off  p_nominal_unit=Pa  p_nominal_value=1  U_m_specify=off  U_m_priority=High  U_m=0 m^3/s  U_m_nominal_specify=off  U_m_nominal_unit=m^3/s  U_m_nominal_value=1
      settings: SourceProductName=Acoustical  InternalSimscapePortConfiguration="{\"Bottom\":[],\"Left\":[{\"id\":\"pp\",\"label\":\"+\",\"type\":\"acoustical.acoustical\"}],\"Right\":[{\"id\":\"nn\",\"label\":\"-\",\"type\":\"acoustical.acoustical\"}],\"Top\":[]}"
  Inertance34 : acoustical_lib/Acoustical Elements/Inertance  m=ac.ho.L(23) Pa*s^2/m^3  r_m=0 Pa/(m^3/s)  g_m=1e-12 m^3/(Pa*s)  u_specify=off  u_priority=None  u=0 m^3/s  u_nominal_specify=off  u_nominal_unit=m^3/s  u_nominal_value=1  p_specify=off  p_priority=None  p=0 Pa  p_nominal_specify=off  p_nominal_unit=Pa  p_nominal_value=1  U_m_specify=off  U_m_priority=High  U_m=0 m^3/s  U_m_nominal_specify=off  U_m_nominal_unit=m^3/s  U_m_nominal_value=1
      settings: SourceProductName=Acoustical  InternalSimscapePortConfiguration="{\"Bottom\":[],\"Left\":[{\"id\":\"pp\",\"label\":\"+\",\"type\":\"acoustical.acoustical\"}],\"Right\":[{\"id\":\"nn\",\"label\":\"-\",\"type\":\"acoustical.acoustical\"}],\"Top\":[]}"
  Inertance35 : acoustical_lib/Acoustical Elements/Inertance  m=ac.ho.L(23) Pa*s^2/m^3  r_m=0 Pa/(m^3/s)  g_m=1e-12 m^3/(Pa*s)  u_specify=off  u_priority=None  u=0 m^3/s  u_nominal_specify=off  u_nominal_unit=m^3/s  u_nominal_value=1  p_specify=off  p_priority=None  p=0 Pa  p_nominal_specify=off  p_nominal_unit=Pa  p_nominal_value=1  U_m_specify=off  U_m_priority=High  U_m=0 m^3/s  U_m_nominal_specify=off  U_m_nominal_unit=m^3/s  U_m_nominal_value=1
      settings: SourceProductName=Acoustical  InternalSimscapePortConfiguration="{\"Bottom\":[],\"Left\":[{\"id\":\"pp\",\"label\":\"+\",\"type\":\"acoustical.acoustical\"}],\"Right\":[{\"id\":\"nn\",\"label\":\"-\",\"type\":\"acoustical.acoustical\"}],\"Top\":[]}"
  Inertance36 : acoustical_lib/Acoustical Elements/Inertance  m=ac.ho.L(24) Pa*s^2/m^3  r_m=0 Pa/(m^3/s)  g_m=1e-12 m^3/(Pa*s)  u_specify=off  u_priority=None  u=0 m^3/s  u_nominal_specify=off  u_nominal_unit=m^3/s  u_nominal_value=1  p_specify=off  p_priority=None  p=0 Pa  p_nominal_specify=off  p_nominal_unit=Pa  p_nominal_value=1  U_m_specify=off  U_m_priority=High  U_m=0 m^3/s  U_m_nominal_specify=off  U_m_nominal_unit=m^3/s  U_m_nominal_value=1
      settings: SourceProductName=Acoustical  InternalSimscapePortConfiguration="{\"Bottom\":[],\"Left\":[{\"id\":\"pp\",\"label\":\"+\",\"type\":\"acoustical.acoustical\"}],\"Right\":[{\"id\":\"nn\",\"label\":\"-\",\"type\":\"acoustical.acoustical\"}],\"Top\":[]}"
  Inertance37 : acoustical_lib/Acoustical Elements/Inertance  m=ac.ho.L(24) Pa*s^2/m^3  r_m=0 Pa/(m^3/s)  g_m=1e-12 m^3/(Pa*s)  u_specify=off  u_priority=None  u=0 m^3/s  u_nominal_specify=off  u_nominal_unit=m^3/s  u_nominal_value=1  p_specify=off  p_priority=None  p=0 Pa  p_nominal_specify=off  p_nominal_unit=Pa  p_nominal_value=1  U_m_specify=off  U_m_priority=High  U_m=0 m^3/s  U_m_nominal_specify=off  U_m_nominal_unit=m^3/s  U_m_nominal_value=1
      settings: SourceProductName=Acoustical  InternalSimscapePortConfiguration="{\"Bottom\":[],\"Left\":[{\"id\":\"pp\",\"label\":\"+\",\"type\":\"acoustical.acoustical\"}],\"Right\":[{\"id\":\"nn\",\"label\":\"-\",\"type\":\"acoustical.acoustical\"}],\"Top\":[]}"
  Inertance38 : acoustical_lib/Acoustical Elements/Inertance  m=ac.ho.L(25) Pa*s^2/m^3  r_m=0 Pa/(m^3/s)  g_m=1e-12 m^3/(Pa*s)  u_specify=off  u_priority=None  u=0 m^3/s  u_nominal_specify=off  u_nominal_unit=m^3/s  u_nominal_value=1  p_specify=off  p_priority=None  p=0 Pa  p_nominal_specify=off  p_nominal_unit=Pa  p_nominal_value=1  U_m_specify=off  U_m_priority=High  U_m=0 m^3/s  U_m_nominal_specify=off  U_m_nominal_unit=m^3/s  U_m_nominal_value=1
      settings: SourceProductName=Acoustical  InternalSimscapePortConfiguration="{\"Bottom\":[],\"Left\":[{\"id\":\"pp\",\"label\":\"+\",\"type\":\"acoustical.acoustical\"}],\"Right\":[{\"id\":\"nn\",\"label\":\"-\",\"type\":\"acoustical.acoustical\"}],\"Top\":[]}"
  Inertance39 : acoustical_lib/Acoustical Elements/Inertance  m=ac.ho.L(25) Pa*s^2/m^3  r_m=0 Pa/(m^3/s)  g_m=1e-12 m^3/(Pa*s)  u_specify=off  u_priority=None  u=0 m^3/s  u_nominal_specify=off  u_nominal_unit=m^3/s  u_nominal_value=1  p_specify=off  p_priority=None  p=0 Pa  p_nominal_specify=off  p_nominal_unit=Pa  p_nominal_value=1  U_m_specify=off  U_m_priority=High  U_m=0 m^3/s  U_m_nominal_specify=off  U_m_nominal_unit=m^3/s  U_m_nominal_value=1
      settings: SourceProductName=Acoustical  InternalSimscapePortConfiguration="{\"Bottom\":[],\"Left\":[{\"id\":\"pp\",\"label\":\"+\",\"type\":\"acoustical.acoustical\"}],\"Right\":[{\"id\":\"nn\",\"label\":\"-\",\"type\":\"acoustical.acoustical\"}],\"Top\":[]}"
  Inertance4 : acoustical_lib/Acoustical Elements/Inertance  m=ac.ho.L(3) Pa*s^2/m^3  r_m=0 Pa/(m^3/s)  g_m=1e-12 m^3/(Pa*s)  u_specify=off  u_priority=None  u=0 m^3/s  u_nominal_specify=off  u_nominal_unit=m^3/s  u_nominal_value=1  p_specify=off  p_priority=None  p=0 Pa  p_nominal_specify=off  p_nominal_unit=Pa  p_nominal_value=1  U_m_specify=off  U_m_priority=High  U_m=0 m^3/s  U_m_nominal_specify=off  U_m_nominal_unit=m^3/s  U_m_nominal_value=1
      settings: SourceProductName=Acoustical  InternalSimscapePortConfiguration="{\"Bottom\":[],\"Left\":[{\"id\":\"pp\",\"label\":\"+\",\"type\":\"acoustical.acoustical\"}],\"Right\":[{\"id\":\"nn\",\"label\":\"-\",\"type\":\"acoustical.acoustical\"}],\"Top\":[]}"
  Inertance40 : acoustical_lib/Acoustical Elements/Inertance  m=ac.ho.L(26) Pa*s^2/m^3  r_m=0 Pa/(m^3/s)  g_m=1e-12 m^3/(Pa*s)  u_specify=off  u_priority=None  u=0 m^3/s  u_nominal_specify=off  u_nominal_unit=m^3/s  u_nominal_value=1  p_specify=off  p_priority=None  p=0 Pa  p_nominal_specify=off  p_nominal_unit=Pa  p_nominal_value=1  U_m_specify=off  U_m_priority=High  U_m=0 m^3/s  U_m_nominal_specify=off  U_m_nominal_unit=m^3/s  U_m_nominal_value=1
      settings: SourceProductName=Acoustical  InternalSimscapePortConfiguration="{\"Bottom\":[],\"Left\":[{\"id\":\"pp\",\"label\":\"+\",\"type\":\"acoustical.acoustical\"}],\"Right\":[{\"id\":\"nn\",\"label\":\"-\",\"type\":\"acoustical.acoustical\"}],\"Top\":[]}"
  Inertance41 : acoustical_lib/Acoustical Elements/Inertance  m=ac.ho.L(26) Pa*s^2/m^3  r_m=0 Pa/(m^3/s)  g_m=1e-12 m^3/(Pa*s)  u_specify=off  u_priority=None  u=0 m^3/s  u_nominal_specify=off  u_nominal_unit=m^3/s  u_nominal_value=1  p_specify=off  p_priority=None  p=0 Pa  p_nominal_specify=off  p_nominal_unit=Pa  p_nominal_value=1  U_m_specify=off  U_m_priority=High  U_m=0 m^3/s  U_m_nominal_specify=off  U_m_nominal_unit=m^3/s  U_m_nominal_value=1
      settings: SourceProductName=Acoustical  InternalSimscapePortConfiguration="{\"Bottom\":[],\"Left\":[{\"id\":\"pp\",\"label\":\"+\",\"type\":\"acoustical.acoustical\"}],\"Right\":[{\"id\":\"nn\",\"label\":\"-\",\"type\":\"acoustical.acoustical\"}],\"Top\":[]}"
  Inertance42 : acoustical_lib/Acoustical Elements/Inertance  m=ac.ho.L(18) Pa*s^2/m^3  r_m=0 Pa/(m^3/s)  g_m=1e-12 m^3/(Pa*s)  u_specify=off  u_priority=None  u=0 m^3/s  u_nominal_specify=off  u_nominal_unit=m^3/s  u_nominal_value=1  p_specify=off  p_priority=None  p=0 Pa  p_nominal_specify=off  p_nominal_unit=Pa  p_nominal_value=1  U_m_specify=off  U_m_priority=High  U_m=0 m^3/s  U_m_nominal_specify=off  U_m_nominal_unit=m^3/s  U_m_nominal_value=1
      settings: SourceProductName=Acoustical  InternalSimscapePortConfiguration="{\"Bottom\":[],\"Left\":[{\"id\":\"pp\",\"label\":\"+\",\"type\":\"acoustical.acoustical\"}],\"Right\":[{\"id\":\"nn\",\"label\":\"-\",\"type\":\"acoustical.acoustical\"}],\"Top\":[]}"
  Inertance43 : acoustical_lib/Acoustical Elements/Inertance  m=ac.ho.L(27) Pa*s^2/m^3  r_m=0 Pa/(m^3/s)  g_m=1e-12 m^3/(Pa*s)  u_specify=off  u_priority=None  u=0 m^3/s  u_nominal_specify=off  u_nominal_unit=m^3/s  u_nominal_value=1  p_specify=off  p_priority=None  p=0 Pa  p_nominal_specify=off  p_nominal_unit=Pa  p_nominal_value=1  U_m_specify=off  U_m_priority=High  U_m=0 m^3/s  U_m_nominal_specify=off  U_m_nominal_unit=m^3/s  U_m_nominal_value=1
      settings: SourceProductName=Acoustical  InternalSimscapePortConfiguration="{\"Bottom\":[],\"Left\":[{\"id\":\"pp\",\"label\":\"+\",\"type\":\"acoustical.acoustical\"}],\"Right\":[{\"id\":\"nn\",\"label\":\"-\",\"type\":\"acoustical.acoustical\"}],\"Top\":[]}"
  Inertance44 : acoustical_lib/Acoustical Elements/Inertance  m=ac.ho.L(27) Pa*s^2/m^3  r_m=0 Pa/(m^3/s)  g_m=1e-12 m^3/(Pa*s)  u_specify=off  u_priority=None  u=0 m^3/s  u_nominal_specify=off  u_nominal_unit=m^3/s  u_nominal_value=1  p_specify=off  p_priority=None  p=0 Pa  p_nominal_specify=off  p_nominal_unit=Pa  p_nominal_value=1  U_m_specify=off  U_m_priority=High  U_m=0 m^3/s  U_m_nominal_specify=off  U_m_nominal_unit=m^3/s  U_m_nominal_value=1
      settings: SourceProductName=Acoustical  InternalSimscapePortConfiguration="{\"Bottom\":[],\"Left\":[{\"id\":\"pp\",\"label\":\"+\",\"type\":\"acoustical.acoustical\"}],\"Right\":[{\"id\":\"nn\",\"label\":\"-\",\"type\":\"acoustical.acoustical\"}],\"Top\":[]}"
  Inertance45 : acoustical_lib/Acoustical Elements/Inertance  m=ac.ho.L(19) Pa*s^2/m^3  r_m=0 Pa/(m^3/s)  g_m=1e-12 m^3/(Pa*s)  u_specify=off  u_priority=None  u=0 m^3/s  u_nominal_specify=off  u_nominal_unit=m^3/s  u_nominal_value=1  p_specify=off  p_priority=None  p=0 Pa  p_nominal_specify=off  p_nominal_unit=Pa  p_nominal_value=1  U_m_specify=off  U_m_priority=High  U_m=0 m^3/s  U_m_nominal_specify=off  U_m_nominal_unit=m^3/s  U_m_nominal_value=1
      settings: SourceProductName=Acoustical  InternalSimscapePortConfiguration="{\"Bottom\":[],\"Left\":[{\"id\":\"pp\",\"label\":\"+\",\"type\":\"acoustical.acoustical\"}],\"Right\":[{\"id\":\"nn\",\"label\":\"-\",\"type\":\"acoustical.acoustical\"}],\"Top\":[]}"
  Inertance46 : acoustical_lib/Acoustical Elements/Inertance  m=ac.ho.L(19) Pa*s^2/m^3  r_m=0 Pa/(m^3/s)  g_m=1e-12 m^3/(Pa*s)  u_specify=off  u_priority=None  u=0 m^3/s  u_nominal_specify=off  u_nominal_unit=m^3/s  u_nominal_value=1  p_specify=off  p_priority=None  p=0 Pa  p_nominal_specify=off  p_nominal_unit=Pa  p_nominal_value=1  U_m_specify=off  U_m_priority=High  U_m=0 m^3/s  U_m_nominal_specify=off  U_m_nominal_unit=m^3/s  U_m_nominal_value=1
      settings: SourceProductName=Acoustical  InternalSimscapePortConfiguration="{\"Bottom\":[],\"Left\":[{\"id\":\"pp\",\"label\":\"+\",\"type\":\"acoustical.acoustical\"}],\"Right\":[{\"id\":\"nn\",\"label\":\"-\",\"type\":\"acoustical.acoustical\"}],\"Top\":[]}"
  Inertance47 : acoustical_lib/Acoustical Elements/Inertance  m=ac.ho.L(18) Pa*s^2/m^3  r_m=0 Pa/(m^3/s)  g_m=1e-12 m^3/(Pa*s)  u_specify=off  u_priority=None  u=0 m^3/s  u_nominal_specify=off  u_nominal_unit=m^3/s  u_nominal_value=1  p_specify=off  p_priority=None  p=0 Pa  p_nominal_specify=off  p_nominal_unit=Pa  p_nominal_value=1  U_m_specify=off  U_m_priority=High  U_m=0 m^3/s  U_m_nominal_specify=off  U_m_nominal_unit=m^3/s  U_m_nominal_value=1
      settings: SourceProductName=Acoustical  InternalSimscapePortConfiguration="{\"Bottom\":[],\"Left\":[{\"id\":\"pp\",\"label\":\"+\",\"type\":\"acoustical.acoustical\"}],\"Right\":[{\"id\":\"nn\",\"label\":\"-\",\"type\":\"acoustical.acoustical\"}],\"Top\":[]}"
  Inertance48 : acoustical_lib/Acoustical Elements/Inertance  m=ac.ho.L(20) Pa*s^2/m^3  r_m=0 Pa/(m^3/s)  g_m=1e-12 m^3/(Pa*s)  u_specify=off  u_priority=None  u=0 m^3/s  u_nominal_specify=off  u_nominal_unit=m^3/s  u_nominal_value=1  p_specify=off  p_priority=None  p=0 Pa  p_nominal_specify=off  p_nominal_unit=Pa  p_nominal_value=1  U_m_specify=off  U_m_priority=High  U_m=0 m^3/s  U_m_nominal_specify=off  U_m_nominal_unit=m^3/s  U_m_nominal_value=1
      settings: SourceProductName=Acoustical  InternalSimscapePortConfiguration="{\"Bottom\":[],\"Left\":[{\"id\":\"pp\",\"label\":\"+\",\"type\":\"acoustical.acoustical\"}],\"Right\":[{\"id\":\"nn\",\"label\":\"-\",\"type\":\"acoustical.acoustical\"}],\"Top\":[]}"
  Inertance49 : acoustical_lib/Acoustical Elements/Inertance  m=ac.ho.L(20) Pa*s^2/m^3  r_m=0 Pa/(m^3/s)  g_m=1e-12 m^3/(Pa*s)  u_specify=off  u_priority=None  u=0 m^3/s  u_nominal_specify=off  u_nominal_unit=m^3/s  u_nominal_value=1  p_specify=off  p_priority=None  p=0 Pa  p_nominal_specify=off  p_nominal_unit=Pa  p_nominal_value=1  U_m_specify=off  U_m_priority=High  U_m=0 m^3/s  U_m_nominal_specify=off  U_m_nominal_unit=m^3/s  U_m_nominal_value=1
      settings: SourceProductName=Acoustical  InternalSimscapePortConfiguration="{\"Bottom\":[],\"Left\":[{\"id\":\"pp\",\"label\":\"+\",\"type\":\"acoustical.acoustical\"}],\"Right\":[{\"id\":\"nn\",\"label\":\"-\",\"type\":\"acoustical.acoustical\"}],\"Top\":[]}"
  Inertance5 : acoustical_lib/Acoustical Elements/Inertance  m=ac.ho.L(3) Pa*s^2/m^3  r_m=0 Pa/(m^3/s)  g_m=1e-12 m^3/(Pa*s)  u_specify=off  u_priority=None  u=0 m^3/s  u_nominal_specify=off  u_nominal_unit=m^3/s  u_nominal_value=1  p_specify=off  p_priority=None  p=0 Pa  p_nominal_specify=off  p_nominal_unit=Pa  p_nominal_value=1  U_m_specify=off  U_m_priority=High  U_m=0 m^3/s  U_m_nominal_specify=off  U_m_nominal_unit=m^3/s  U_m_nominal_value=1
      settings: SourceProductName=Acoustical  InternalSimscapePortConfiguration="{\"Bottom\":[],\"Left\":[{\"id\":\"pp\",\"label\":\"+\",\"type\":\"acoustical.acoustical\"}],\"Right\":[{\"id\":\"nn\",\"label\":\"-\",\"type\":\"acoustical.acoustical\"}],\"Top\":[]}"
  Inertance50 : acoustical_lib/Acoustical Elements/Inertance  m=ac.ho.L(21) Pa*s^2/m^3  r_m=0 Pa/(m^3/s)  g_m=1e-12 m^3/(Pa*s)  u_specify=off  u_priority=None  u=0 m^3/s  u_nominal_specify=off  u_nominal_unit=m^3/s  u_nominal_value=1  p_specify=off  p_priority=None  p=0 Pa  p_nominal_specify=off  p_nominal_unit=Pa  p_nominal_value=1  U_m_specify=off  U_m_priority=High  U_m=0 m^3/s  U_m_nominal_specify=off  U_m_nominal_unit=m^3/s  U_m_nominal_value=1
      settings: SourceProductName=Acoustical  InternalSimscapePortConfiguration="{\"Bottom\":[],\"Left\":[{\"id\":\"pp\",\"label\":\"+\",\"type\":\"acoustical.acoustical\"}],\"Right\":[{\"id\":\"nn\",\"label\":\"-\",\"type\":\"acoustical.acoustical\"}],\"Top\":[]}"
  Inertance51 : acoustical_lib/Acoustical Elements/Inertance  m=ac.ho.L(21) Pa*s^2/m^3  r_m=0 Pa/(m^3/s)  g_m=1e-12 m^3/(Pa*s)  u_specify=off  u_priority=None  u=0 m^3/s  u_nominal_specify=off  u_nominal_unit=m^3/s  u_nominal_value=1  p_specify=off  p_priority=None  p=0 Pa  p_nominal_specify=off  p_nominal_unit=Pa  p_nominal_value=1  U_m_specify=off  U_m_priority=High  U_m=0 m^3/s  U_m_nominal_specify=off  U_m_nominal_unit=m^3/s  U_m_nominal_value=1
      settings: SourceProductName=Acoustical  InternalSimscapePortConfiguration="{\"Bottom\":[],\"Left\":[{\"id\":\"pp\",\"label\":\"+\",\"type\":\"acoustical.acoustical\"}],\"Right\":[{\"id\":\"nn\",\"label\":\"-\",\"type\":\"acoustical.acoustical\"}],\"Top\":[]}"
  Inertance52 : acoustical_lib/Acoustical Elements/Inertance  m=ac.ho.L(22) Pa*s^2/m^3  r_m=0 Pa/(m^3/s)  g_m=1e-12 m^3/(Pa*s)  u_specify=off  u_priority=None  u=0 m^3/s  u_nominal_specify=off  u_nominal_unit=m^3/s  u_nominal_value=1  p_specify=off  p_priority=None  p=0 Pa  p_nominal_specify=off  p_nominal_unit=Pa  p_nominal_value=1  U_m_specify=off  U_m_priority=High  U_m=0 m^3/s  U_m_nominal_specify=off  U_m_nominal_unit=m^3/s  U_m_nominal_value=1
      settings: SourceProductName=Acoustical  InternalSimscapePortConfiguration="{\"Bottom\":[],\"Left\":[{\"id\":\"pp\",\"label\":\"+\",\"type\":\"acoustical.acoustical\"}],\"Right\":[{\"id\":\"nn\",\"label\":\"-\",\"type\":\"acoustical.acoustical\"}],\"Top\":[]}"
  Inertance53 : acoustical_lib/Acoustical Elements/Inertance  m=ac.ho.L(22) Pa*s^2/m^3  r_m=0 Pa/(m^3/s)  g_m=1e-12 m^3/(Pa*s)  u_specify=off  u_priority=None  u=0 m^3/s  u_nominal_specify=off  u_nominal_unit=m^3/s  u_nominal_value=1  p_specify=off  p_priority=None  p=0 Pa  p_nominal_specify=off  p_nominal_unit=Pa  p_nominal_value=1  U_m_specify=off  U_m_priority=High  U_m=0 m^3/s  U_m_nominal_specify=off  U_m_nominal_unit=m^3/s  U_m_nominal_value=1
      settings: SourceProductName=Acoustical  InternalSimscapePortConfiguration="{\"Bottom\":[],\"Left\":[{\"id\":\"pp\",\"label\":\"+\",\"type\":\"acoustical.acoustical\"}],\"Right\":[{\"id\":\"nn\",\"label\":\"-\",\"type\":\"acoustical.acoustical\"}],\"Top\":[]}"
  Inertance6 : acoustical_lib/Acoustical Elements/Inertance  m=ac.ho.L(4) Pa*s^2/m^3  r_m=0 Pa/(m^3/s)  g_m=1e-12 m^3/(Pa*s)  u_specify=off  u_priority=None  u=0 m^3/s  u_nominal_specify=off  u_nominal_unit=m^3/s  u_nominal_value=1  p_specify=off  p_priority=None  p=0 Pa  p_nominal_specify=off  p_nominal_unit=Pa  p_nominal_value=1  U_m_specify=off  U_m_priority=High  U_m=0 m^3/s  U_m_nominal_specify=off  U_m_nominal_unit=m^3/s  U_m_nominal_value=1
      settings: SourceProductName=Acoustical  InternalSimscapePortConfiguration="{\"Bottom\":[],\"Left\":[{\"id\":\"pp\",\"label\":\"+\",\"type\":\"acoustical.acoustical\"}],\"Right\":[{\"id\":\"nn\",\"label\":\"-\",\"type\":\"acoustical.acoustical\"}],\"Top\":[]}"
  Inertance7 : acoustical_lib/Acoustical Elements/Inertance  m=ac.ho.L(4) Pa*s^2/m^3  r_m=0 Pa/(m^3/s)  g_m=1e-12 m^3/(Pa*s)  u_specify=off  u_priority=None  u=0 m^3/s  u_nominal_specify=off  u_nominal_unit=m^3/s  u_nominal_value=1  p_specify=off  p_priority=None  p=0 Pa  p_nominal_specify=off  p_nominal_unit=Pa  p_nominal_value=1  U_m_specify=off  U_m_priority=High  U_m=0 m^3/s  U_m_nominal_specify=off  U_m_nominal_unit=m^3/s  U_m_nominal_value=1
      settings: SourceProductName=Acoustical  InternalSimscapePortConfiguration="{\"Bottom\":[],\"Left\":[{\"id\":\"pp\",\"label\":\"+\",\"type\":\"acoustical.acoustical\"}],\"Right\":[{\"id\":\"nn\",\"label\":\"-\",\"type\":\"acoustical.acoustical\"}],\"Top\":[]}"
  Inertance8 : acoustical_lib/Acoustical Elements/Inertance  m=ac.ho.L(5) Pa*s^2/m^3  r_m=0 Pa/(m^3/s)  g_m=1e-12 m^3/(Pa*s)  u_specify=off  u_priority=None  u=0 m^3/s  u_nominal_specify=off  u_nominal_unit=m^3/s  u_nominal_value=1  p_specify=off  p_priority=None  p=0 Pa  p_nominal_specify=off  p_nominal_unit=Pa  p_nominal_value=1  U_m_specify=off  U_m_priority=High  U_m=0 m^3/s  U_m_nominal_specify=off  U_m_nominal_unit=m^3/s  U_m_nominal_value=1
      settings: SourceProductName=Acoustical  InternalSimscapePortConfiguration="{\"Bottom\":[],\"Left\":[{\"id\":\"pp\",\"label\":\"+\",\"type\":\"acoustical.acoustical\"}],\"Right\":[{\"id\":\"nn\",\"label\":\"-\",\"type\":\"acoustical.acoustical\"}],\"Top\":[]}"
  Inertance9 : acoustical_lib/Acoustical Elements/Inertance  m=ac.ho.L(5) Pa*s^2/m^3  r_m=0 Pa/(m^3/s)  g_m=1e-12 m^3/(Pa*s)  u_specify=off  u_priority=None  u=0 m^3/s  u_nominal_specify=off  u_nominal_unit=m^3/s  u_nominal_value=1  p_specify=off  p_priority=None  p=0 Pa  p_nominal_specify=off  p_nominal_unit=Pa  p_nominal_value=1  U_m_specify=off  U_m_priority=High  U_m=0 m^3/s  U_m_nominal_specify=off  U_m_nominal_unit=m^3/s  U_m_nominal_value=1
      settings: SourceProductName=Acoustical  InternalSimscapePortConfiguration="{\"Bottom\":[],\"Left\":[{\"id\":\"pp\",\"label\":\"+\",\"type\":\"acoustical.acoustical\"}],\"Right\":[{\"id\":\"nn\",\"label\":\"-\",\"type\":\"acoustical.acoustical\"}],\"Top\":[]}"
  1+ : PMIOPort  Side=Left
  1- : PMIOPort  Port=2  Side=Left
  2+ : PMIOPort  Port=3  Side=Right
  2- : PMIOPort  Port=4  Side=Right
  connections:
  Inertance/LConn1 -- 1+/RConn1
  Inertance9/RConn1 -- Inertance10/LConn1
  Inertance13/RConn1 -- Inertance14/LConn1
  2+/RConn1 -- Inertance44/RConn1
  Compliance6/LConn1 -- Inertance13/LConn1 -- Inertance12/RConn1
  Compliance4/LConn1 -- Inertance9/LConn1 -- Inertance8/RConn1
  Inertance47/RConn1 -- Inertance45/LConn1
  Inertance5/RConn1 -- Inertance6/LConn1
  Inertance49/RConn1 -- Inertance50/LConn1
  Inertance41/RConn1 -- Inertance43/LConn1
  Inertance53/RConn1 -- Inertance34/LConn1
  Compliance21/LConn1 -- Inertance53/LConn1 -- Inertance52/RConn1
  Compliance26/LConn1 -- Inertance44/LConn1 -- Inertance43/RConn1
  Compliance7/LConn1 -- Inertance15/LConn1 -- Inertance14/RConn1
  Compliance22/LConn1 -- Inertance35/LConn1 -- Inertance34/RConn1
  Inertance52/LConn1 -- Inertance51/RConn1
  Compliance19/LConn1 -- Inertance49/LConn1 -- Inertance48/RConn1
  Inertance17/RConn1 -- Inertance24/LConn1
  Inertance19/RConn1 -- Inertance20/LConn1
  Inertance35/RConn1 -- Inertance36/LConn1
  Compliance1/RConn1 -- Compliance6/RConn1 -- Compliance7/RConn1 -- Compliance8/RConn1 -- Compliance9/RConn1 -- Compliance10/RConn1 -- Compliance11/RConn1 -- Compliance12/RConn1 -- Compliance13/RConn1 -- Compliance14/RConn1 -- Compliance15/RConn1 -- Compliance16/RConn1 -- Compliance17/RConn1 -- 2-/RConn1 -- Compliance26/RConn1 -- Compliance25/RConn1 -- Compliance24/RConn1 -- Compliance23/RConn1 -- Compliance22/RConn1 -- Compliance21/RConn1 -- Compliance20/RConn1 -- Compliance19/RConn1 -- Compliance18/RConn1 -- Compliance5/RConn1 -- Compliance4/RConn1 -- Compliance3/RConn1 -- Compliance2/RConn1 -- 1-/RConn1 -- Compliance/RConn1
  Inertance25/RConn1 -- Inertance26/LConn1
  Compliance20/LConn1 -- Inertance51/LConn1 -- Inertance50/RConn1
  Compliance25/LConn1 -- Inertance41/LConn1 -- Inertance40/RConn1
  Compliance10/LConn1 -- Inertance27/LConn1 -- Inertance26/RConn1
  Inertance30/LConn1 -- Inertance29/RConn1
  Inertance31/RConn1 -- Inertance18/LConn1
  Inertance21/RConn1 -- Inertance22/LConn1
  Compliance9/LConn1 -- Inertance25/LConn1 -- Inertance24/RConn1
  Compliance11/LConn1 -- Inertance29/LConn1 -- Inertance28/RConn1
  Inertance37/RConn1 -- Inertance38/LConn1
  Compliance8/LConn1 -- Inertance17/LConn1 -- Inertance16/RConn1
  Inertance8/LConn1 -- Inertance7/RConn1
  Inertance3/RConn1 -- Inertance4/LConn1
  Compliance15/LConn1 -- Inertance23/LConn1 -- Inertance22/RConn1
  Compliance24/LConn1 -- Inertance39/LConn1 -- Inertance38/RConn1
  Compliance3/LConn1 -- Inertance7/LConn1 -- Inertance6/RConn1
  Inertance48/LConn1 -- Inertance46/RConn1
  Inertance23/RConn1 -- Inertance32/LConn1
  Compliance/LConn1 -- Inertance1/LConn1 -- Inertance/RConn1
  Inertance33/RConn1 -- Inertance42/LConn1
  Inertance1/RConn1 -- Inertance2/LConn1
  Inertance27/RConn1 -- Inertance28/LConn1
  Inertance39/RConn1 -- Inertance40/LConn1
  Compliance23/LConn1 -- Inertance37/LConn1 -- Inertance36/RConn1
  Compliance5/LConn1 -- Inertance11/LConn1 -- Inertance10/RConn1
  Compliance17/LConn1 -- Inertance47/LConn1 -- Inertance42/RConn1
  Inertance15/RConn1 -- Inertance16/LConn1
  Compliance2/LConn1 -- Inertance5/LConn1 -- Inertance4/RConn1
  Compliance16/LConn1 -- Inertance33/LConn1 -- Inertance32/RConn1
  Compliance1/LConn1 -- Inertance3/LConn1 -- Inertance2/RConn1
  Compliance12/LConn1 -- Inertance31/LConn1 -- Inertance30/RConn1
  Inertance11/RConn1 -- Inertance12/LConn1
  Compliance18/LConn1 -- Inertance46/LConn1 -- Inertance45/RConn1
  Compliance14/LConn1 -- Inertance21/LConn1 -- Inertance20/RConn1
  Compliance13/LConn1 -- Inertance19/LConn1 -- Inertance18/RConn1
